simulink model "AlgebricLoop"  (R2020a)
settings: Solver=VariableStepAuto  StartTime=0.0  StopTime=10.0  RelTol=1e-3
settings Model: Creator=ashok  LastModifiedBy=ashok

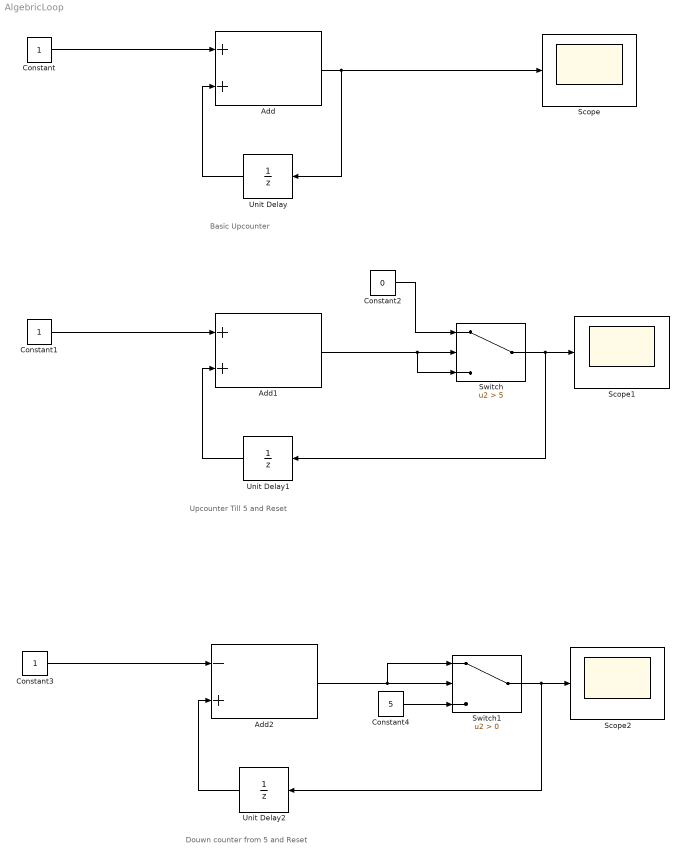
== system AlgebricLoop ==
  note: Basic Upcounter
  note: Upcounter Till 5 and Reset
  note: Douwn counter from 5 and Reset
  Add : Sum
  Add1 : Sum
  Add2 : Sum  Inputs=-+
  Constant : Constant
  Constant1 : Constant
  Constant2 : Constant  Value=0
  Constant3 : Constant
  Constant4 : Constant  Value=5
  Scope : Scope
  Scope1 : Scope
  Scope2 : Scope
  Switch : Switch  Criteria=u2 > Threshold  Threshold=5
  Switch1 : Switch  Criteria=u2 > Threshold
  Unit Delay : UnitDelay  SampleTime=-1  HasFrameUpgradeWarning=on
  Unit Delay1 : UnitDelay  SampleTime=-1  HasFrameUpgradeWarning=on
  Unit Delay2 : UnitDelay  SampleTime=-1  HasFrameUpgradeWarning=on
  wires:
  Constant/1 -> Add/1
  Add/1 -> Scope/1, Unit Delay/1
  Unit Delay/1 -> Add/2
  Constant1/1 -> Add1/1
  Unit Delay1/1 -> Add1/2
  Add1/1 -> Switch/3, Switch/2
  Switch/1 -> Unit Delay1/1, Scope1/1
  Constant2/1 -> Switch/1
  Switch1/1 -> Unit Delay2/1, Scope2/1
  Constant3/1 -> Add2/1
  Unit Delay2/1 -> Add2/2
  Add2/1 -> Switch1/1, Switch1/2
  Constant4/1 -> Switch1/3
